simulink model "Model_with_Opt_Cntrl_ver3_US"  (R2024a)
settings: Solver=FixedStepAuto  StartTime=0.0  StopTime=31  FixedStep=h  RelTol=1e-3
values from neighbouring files (symbols this model uses):
  alpha = 0.5    [gamma1.m]
  beta = 1.907e-06    [gamma1.m]
  delta = delta_vect(i)    [gamma1.m]
  epsilon = 0.25    [gamma1.m]
  eta = 0.03974    [gamma1.m]
  gamma = 0.1054    [gamma1.m]
  h = 0.1    [gamma1.m]
  Lambda = 1.139425534473202e+03    (= 1139.42553447)    [gamma1.m]
  mu = 0.5669    [gamma1.m]
  mu_0 = 0.2    [gamma1.m]
  p_0 = 0.28555    [gamma1.m]
  p_max = 0.74    [gamma1.m]
  xi = 0.90    (= 0.9)    [gamma1.m]
undefined symbols (not defined in the file or in its folder): m1, m2, m3, n1, n2, n3
settings Model: Creator=HEV-Laptop  LastModifiedBy=nuzhatnuarikhanrivu
settings SolverCC: AlgebraicLoopSolver=TrustRegion
settings DataIOCC: OutputOption=AdditionalOutputTimes  OutputTimes=SDO_OutputTimes  ReturnWorkspaceOutputsName=SDOSimTest_Log
settings DebuggingCC: UnconnectedInputMsg=warning  UnconnectedOutputMsg=warning  UnconnectedLineMsg=warning
settings ModelReferenceCC: EnableRefExpFcnMdlSchedulingChecks=on
settings RTWCC: GPUComputeCapability=3.5

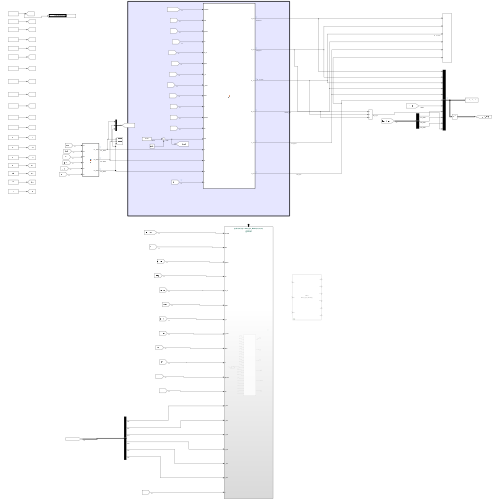
[thumbnail: Simulink's stored preview of the top-level diagram]
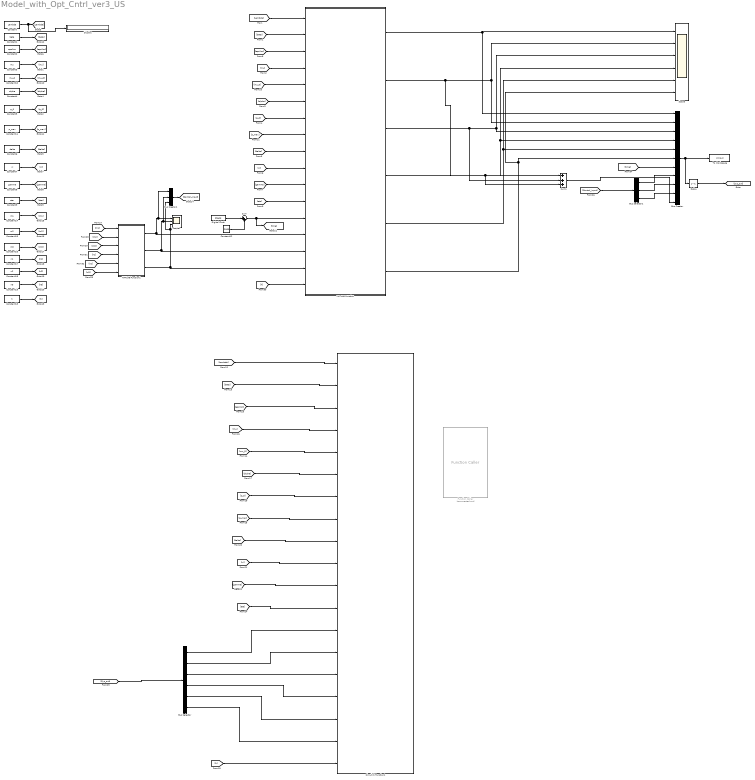
== system Model_with_Opt_Cntrl_ver3_US ==
  Bus Creator : BusCreator  Inputs=11
  Bus Creator1 : BusCreator  Inputs=3
  Bus Selector : BusSelector  OutputSignals=S,E,I1,I2,T,A
  Bus Selector1 : BusSelector  OutputSignals=u1_final,u2_final,u3_final
  Constant : Constant  Value=Lambda
  Constant1 : Constant  Value=beta
  Constant10 : Constant  Value=mu_0
  Constant11 : Constant  Value=p_max
  Constant12 : Constant  Value=2000
  Constant13 : Constant  Value=h
  Constant14 : Constant  Value=m1
  Constant15 : Constant  Value=m2
  Constant16 : Constant  Value=m3
  Constant17 : Constant  Value=n1
  Constant18 : Constant  Value=n2
  Constant19 : Constant  Value=n3
  Constant2 : Constant  Value=epsilon
  Constant3 : Constant  Value=mu
  Constant4 : Constant  Value=alpha
  Constant5 : Constant  Value=p_0
  Constant6 : Constant  Value=delta
  Constant7 : Constant  Value=xi
  Constant8 : Constant  Value=gamma
  Constant9 : Constant  Value=eta
  Delay : Delay  DelayLength=1
  Digital Clock : DigitalClock  SampleTime=h
  Display : Display
  Function Caller : FunctionCaller  Commented=on  FunctionPrototype=[S,E,I1,I2,T,A] = Aids_Sys_Model(u1,u2,u3)  InputArgumentSpecifications=<Enter example>  OutputArgumentSpecifications=<Enter example>
  MATLAB Function : MATLAB Function  TreatAsAtomicUnit=on
  MATLAB Function1 : MATLAB Function  TreatAsAtomicUnit=on
  Scope : Scope  NumInputPorts=6
  Scope1 : Scope  NumInputPorts=3
  Simulink Function1 : Subsystem  TreatAsAtomicUnit=on
  Sum : Sum  Inputs=|++
  Sum1 : Sum  Inputs=+++
  To Workspace : ToWorkspace  VariableName=simout  SaveFormat=Timeseries  SampleTime=-1
  wires:
  [Lambda] -> MATLAB Function/1(Lambda)
  Constant/1 -> Display/1, [Lambda]
  MATLAB Function/1(S_n1) -> Bus Creator/1, Scope/1  "S"
  MATLAB Function/2(E_n1) -> Sum1/1, Bus Creator/2, Scope/2  "E"
  MATLAB Function/3(I1_n1) -> Bus Creator/3, Scope/3, Sum1/2  "I1"
  Bus Creator/1 -> Delay/1, To Workspace/1
  Constant1/1 -> [beta]
  [beta] -> MATLAB Function/2(beta)
  Constant2/1 -> [epsilon]
  [epsilon] -> MATLAB Function/3(epsilon)
  Constant3/1 -> [mu]
  [mu] -> MATLAB Function/4(mu)
  Constant4/1 -> [alpha]
  [alpha] -> MATLAB Function/6(alpha)
  Constant5/1 -> [p_0]
  [p_0] -> MATLAB Function/7(p_0)
  Constant6/1 -> [delta]
  Constant7/1 -> [xi]
  Constant8/1 -> [gamma]
  [delta] -> MATLAB Function/9(delta)
  [xi] -> MATLAB Function/10(xi)
  [gamma] -> MATLAB Function/11(gamma)
  Constant9/1 -> [eta]
  [eta] -> MATLAB Function/12(eta)
  Constant10/1 -> [mu_0]
  [mu_0] -> MATLAB Function/5(mu_0)
  MATLAB Function/4(I2_n1) -> Sum1/3, Scope/4, Bus Creator/4  "I2"
  MATLAB Function/5(T_n1) -> Scope/5, Bus Creator/5  "T"
  MATLAB Function/6(A_n1) -> Scope/6, Bus Creator/6  "A"
  Constant11/1 -> [p_max]
  [p_max] -> MATLAB Function/8(p_max)
  Sum/1 -> [time], MATLAB Function/13(time)  "time"
  Digital Clock/1 -> Sum/1  "time"
  Constant12/1 -> Sum/2
  [h] -> MATLAB Function/17(h)
  Constant13/1 -> [h]
  MATLAB Function1/2(u2_final) -> Bus Creator1/2, Scope1/2, MATLAB Function/15(u2)
  MATLAB Function1/3(u3_final) -> Bus Creator1/3, Scope1/3, MATLAB Function/16(u3)
  MATLAB Function1/1(u1_final) -> Bus Creator1/1, Scope1/1, MATLAB Function/14(u1)
  [Lambda] -> Simulink Function1/1(Lambda)
  [beta] -> Simulink Function1/2(beta)
  [epsilon] -> Simulink Function1/3(epsilon)
  [mu] -> Simulink Function1/4(mu)
  [mu_0] -> Simulink Function1/5(mu_0)
  [alpha] -> Simulink Function1/6(alpha)
  [p_0] -> Simulink Function1/7(p_0)
  [p_max] -> Simulink Function1/8(p_max)
  [delta] -> Simulink Function1/9(delta)
  [xi] -> Simulink Function1/10(xi)
  [gamma] -> Simulink Function1/11(gamma)
  [eta] -> Simulink Function1/12(eta)
  [h] -> Simulink Function1/19(h)
  [Sys_out] -> Bus Selector/1
  Bus Selector/3 -> Simulink Function1/15(I1_init)  "<I1>"
  Bus Selector/2 -> Simulink Function1/14(E_init)  "<E>"
  Bus Selector/4 -> Simulink Function1/16(I2_init)  "<I2>"
  Bus Selector/1 -> Simulink Function1/13(S_init)  "<S>"
  Bus Selector/5 -> Simulink Function1/17(T_init)  "<T>"
  Bus Selector/6 -> Simulink Function1/18(A_init)  "<A>"
  Delay/1 -> [Sys_out]
  Bus Creator1/1 -> [Control_input]
  Constant14/1 -> [m1]
  Constant15/1 -> [m2]
  Constant16/1 -> [m3]
  Constant17/1 -> [n1]
  Constant18/1 -> [n2]
  Constant19/1 -> [n3]
  [m1] -> MATLAB Function1/1(m1)
  [m2] -> MATLAB Function1/2(m2)
  [m3] -> MATLAB Function1/3(m3)
  [n1] -> MATLAB Function1/4(n1)
  [n2] -> MATLAB Function1/5(n2)
  [n3] -> MATLAB Function1/6(n3)
  [Control_input] -> Bus Selector1/1
  [time] -> Bus Creator/7
  Bus Selector1/1 -> Bus Creator/8  "<u1_final>"
  Bus Selector1/2 -> Bus Creator/9  "<u2_final>"
  Bus Selector1/3 -> Bus Creator/10  "<u3_final>"
  Sum1/1 -> Bus Creator/11  "E_I1_I2"

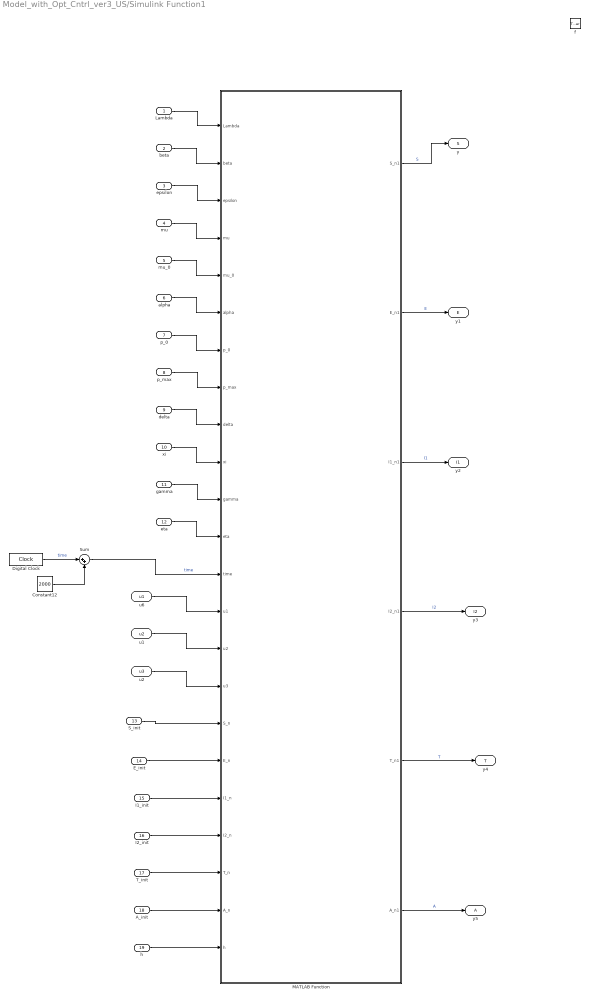
== system Model_with_Opt_Cntrl_ver3_US/Simulink Function1 ==
  Lambda : Inport
  beta : Inport  Port=2
  epsilon : Inport  Port=3
  mu : Inport  Port=4
  mu_0 : Inport  Port=5
  alpha : Inport  Port=6
  p_0 : Inport  Port=7
  p_max : Inport  Port=8
  delta : Inport  Port=9
  xi : Inport  Port=10
  gamma : Inport  Port=11
  eta : Inport  Port=12
  S_init : Inport  Port=13
  E_init : Inport  Port=14
  I1_init : Inport  Port=15
  I2_init : Inport  Port=16
  T_init : Inport  Port=17
  A_init : Inport  Port=18
  h : Inport  Port=19
  f : TriggerPort  TriggerType=function-call  IsSimulinkFunction=on  FunctionName=Aids_Sys_Model  VariantControl=(inherit)
  Constant12 : Constant  Value=2000
  Digital Clock : DigitalClock  SampleTime=-1
  MATLAB Function : MATLAB Function  TreatAsAtomicUnit=on
  Sum : Sum  Inputs=|++
  u6 : ArgIn  DisableCoverage=on  ArgumentName=u1
  u1 : ArgIn  DisableCoverage=on  Port=2  ArgumentName=u2
  u2 : ArgIn  DisableCoverage=on  Port=3  ArgumentName=u3
  y : ArgOut  DisableCoverage=on  ArgumentName=S
  y1 : ArgOut  DisableCoverage=on  Port=2  ArgumentName=E
  y2 : ArgOut  DisableCoverage=on  Port=3  ArgumentName=I1
  y3 : ArgOut  DisableCoverage=on  Port=4  ArgumentName=I2
  y4 : ArgOut  DisableCoverage=on  Port=5  ArgumentName=T
  y5 : ArgOut  DisableCoverage=on  Port=6  ArgumentName=A
  wires:
  Digital Clock/1 -> Sum/1  "time"
  h/1 -> MATLAB Function/23(h)
  mu_0/1 -> MATLAB Function/5(mu_0)
  xi/1 -> MATLAB Function/10(xi)
  mu/1 -> MATLAB Function/4(mu)
  Constant12/1 -> Sum/2
  p_max/1 -> MATLAB Function/8(p_max)
  delta/1 -> MATLAB Function/9(delta)
  Sum/1 -> MATLAB Function/13(time)  "time"
  beta/1 -> MATLAB Function/2(beta)
  eta/1 -> MATLAB Function/12(eta)
  epsilon/1 -> MATLAB Function/3(epsilon)
  p_0/1 -> MATLAB Function/7(p_0)
  alpha/1 -> MATLAB Function/6(alpha)
  Lambda/1 -> MATLAB Function/1(Lambda)
  gamma/1 -> MATLAB Function/11(gamma)
  u6/1 -> MATLAB Function/14(u1)
  u1/1 -> MATLAB Function/15(u2)
  u2/1 -> MATLAB Function/16(u3)
  MATLAB Function/1(S_n1) -> y/1  "S"
  MATLAB Function/2(E_n1) -> y1/1  "E"
  MATLAB Function/3(I1_n1) -> y2/1  "I1"
  MATLAB Function/4(I2_n1) -> y3/1  "I2"
  MATLAB Function/5(T_n1) -> y4/1  "T"
  MATLAB Function/6(A_n1) -> y5/1  "A"
  S_init/1 -> MATLAB Function/17(S_n)
  E_init/1 -> MATLAB Function/18(E_n)
  I1_init/1 -> MATLAB Function/19(I1_n)
  I2_init/1 -> MATLAB Function/20(I2_n)
  T_init/1 -> MATLAB Function/21(T_n)
  A_init/1 -> MATLAB Function/22(A_n)

== matlab function Model_with_Opt_Cntrl_ver3_US/MATLAB Function1 ==
  data: u1_final output; u2_final output; u3_final output; m1 input; m2 input; m3 input; n1 input; n2 input; n3 input
function [u1_final,u2_final,u3_final] = fcn(m1,m2,m3,n1,n2,n3)

u1=linspace(0,1,10);
u2=linspace(0,1,10);
u3=linspace(0,1,10);
% m1,m2,m3,n1,n2,n3
% m1=1;
% m2=1;
% m3=1;
% n1=1;
% n2=0.5;
% n3=1;

cost_mtrx=inf*ones(1000,1);
u1_mtrx=inf*ones(1000,1);
u2_mtrx=inf*ones(1000,1);
u3_mtrx=inf*ones(1000,1);
count=1;
for i=1:length(u1)
    for j=1:length(u2)
        for k=1:length(u3)
            
            [S,E,I1,I2,T,A] = Aids_Sys_Model(u1(i),u2(j),u3(k));
            
            cost=m1*E+m2*I1+m3*I2+(n1/2)*u1(i)^2+(n2/2)*u2(j)^2+(n3/2)*u3(k)^2;
            
            cost_mtrx(count)=cost;
            u1_mtrx(count)=u1(i);
            u2_mtrx(count)=u2(j);
            u3_mtrx(count)=u3(k);
            count=count+1;
            
        end
    end
end

[M,indx]=min(cost_mtrx);

u1_final=u1_mtrx(indx);
u2_final=u2_mtrx(indx);
u3_final=u3_mtrx(indx);

== matlab function Model_with_Opt_Cntrl_ver3_US/Simulink Function1/MATLAB Function ==
  data: Lambda input; beta input; epsilon input; mu input; mu_0 input; alpha input; p_0 input; p_max input; delta input; xi input; gamma input; eta input; time input; u1 input; u2 input; u3 input; S_n input; E_n input; I1_n input; I2_n input; T_n input; A_n input; S_n1 output; E_n1 output; h input; I1_n1 output; I2_n1 output; T_n1 output; A_n1 output
function [S_n1,E_n1,I1_n1,I2_n1,T_n1,A_n1] =fcn(Lambda,beta,epsilon,mu,mu_0,alpha,p_0,p_max,delta,xi,gamma,eta,time,u1,u2,u3,S_n,E_n,I1_n,I2_n,T_n,A_n,h)
% h=1;
% h_m2_n1=0;
% h_f2_n1=0;
% h_f3_n1=0;

% persistent S_n E_n I1_n I2_n T_n A_n
% if isempty(S_n)
%     S_n = 248745348;%924860000;
% end


% if isempty(E_n)
%     E_n = 207095;%770000;
% end

% if isempty(I1_n)
%     I1_n = 73297;%40000;
% end

% if isempty(I2_n)
%     I2_n = 30000;
% end

% if isempty(T_n)
%     T_n = 410;
% end

% if isempty(A_n)
%     A_n = 28235;
% end
a=0.055961;
p=(p_0-p_max)*exp(-a*time)+p_max;


%%S
S_n1=S_n+h*(Lambda-beta*(epsilon*E_n+I2_n)*S_n-mu*S_n);
%%E
E_n1=E_n+h*(beta*(epsilon*E_n+I2_n)*S_n)-(alpha+mu)*E_n-u1*E_n;
%%I1
I1_n1=I1_n+h*(p*alpha*E_n+delta*I2_n-(mu+xi+gamma)*I1_n+u1*E_n++u2*I2_n-u3*I1_n);
%%I2
I2_n1=I2_n+h*((1-p)*alpha*E_n-(delta+gamma+mu)*I2_n-u2*I2_n);
%%T
T_n1=T_n+h*(xi*I1_n-(mu+eta)*T_n)+u3*I1_n;
%%A
A_n1=A_n+h*(gamma*(I1_n+I2_n)+eta*T_n-(mu_0+mu)*A_n);


if(S_n1<0)
    S_n1=0;
end
if(E_n1<0)
    E_n1=0;
end
if(I1_n1<0)
    I1_n1=0;
end
if(I2_n1<0)
    I2_n1=0;
end

if(T_n1<0)
    T_n1=0;
end
if(A_n1<0)
    A_n1=0;
end




S_n=S_n1;
E_n=E_n1;
I1_n=I1_n1;
I2_n=I2_n1;
T_n=T_n1;
A_n=A_n1;

== matlab function Model_with_Opt_Cntrl_ver3_US/MATLAB Function ==
  data: Lambda input; beta input; epsilon input; mu input; mu_0 input; alpha input; p_0 input; p_max input; delta input; xi input; gamma input; eta input; time input; u1 input; u2 input; u3 input; S_n1 output; E_n1 output; h input; I1_n1 output; I2_n1 output; T_n1 output; A_n1 output
function [S_n1,E_n1,I1_n1,I2_n1,T_n1,A_n1] =fcn(Lambda,beta,epsilon,mu,mu_0,alpha,p_0,p_max,delta,xi,gamma,eta,time,u1,u2,u3,h)
% h=1;
% h_m2_n1=0;
% h_f2_n1=0;
% h_f3_n1=0;

persistent S_n E_n I1_n I2_n T_n A_n
if isempty(S_n)
    S_n = 248745348;%924860000;
end


if isempty(E_n)
    E_n = 207095;%770000;
end

if isempty(I1_n)
    I1_n = 73297;%40000;
end

if isempty(I2_n)
    I2_n = 30000;
end

if isempty(T_n)
    T_n = 410;
end

if isempty(A_n)
    A_n = 28235;
end
a=0.055961;
p=(p_0-p_max)*exp(-a*time)+p_max;


%%S
S_n1=S_n+h*(Lambda-beta*(epsilon*E_n+I2_n)*S_n-mu*S_n);
%%E
E_n1=E_n+h*(beta*(epsilon*E_n+I2_n)*S_n)-(alpha+mu)*E_n-u1*E_n;
%%I1
I1_n1=I1_n+h*(p*alpha*E_n+delta*I2_n-(mu+xi+gamma)*I1_n+u1*E_n++u2*I2_n-u3*I1_n);
%%I2
I2_n1=I2_n+h*((1-p)*alpha*E_n-(delta+gamma+mu)*I2_n-u2*I2_n);
%%T
T_n1=T_n+h*(xi*I1_n-(mu+eta)*T_n)+u3*I1_n;
%%A
A_n1=A_n+h*(gamma*(I1_n+I2_n)+eta*T_n-(mu_0+mu)*A_n);


if(S_n1<0)
    S_n1=0;
end
if(E_n1<0)
    E_n1=0;
end
if(I1_n1<0)
    I1_n1=0;
end
if(I2_n1<0)
    I2_n1=0;
end

if(T_n1<0)
    T_n1=0;
end
if(A_n1<0)
    A_n1=0;
end




S_n=S_n1;
E_n=E_n1;
I1_n=I1_n1;
I2_n=I2_n1;
T_n=T_n1;
A_n=A_n1;
